simulink model "CompleteModel"  (R2023a)
settings: Solver=VariableStepAuto  StartTime=0.0  StopTime=10.0  RelTol=1e-3
undefined symbols (not defined in the file): Axle1D, AxleIn, Body, Body_Axle2, Brakes_Axle2_None, Chassis_Axle2, Damper, Damper_Basics, Init, Left, Linear, None, Power, Right, Sedan_Hamba_Parts, ShaftA1, ShaftA2, Spring, Spring_Basics, Vehicle, Visual, X, Y, Z
libraries: sm_lib x272, sm_car_lib x96, fl_lib x69, nesl_utility x51, Driveshaft_ShaftsAll x4, Steer_Rack x3, Differential_Systems x2, sdl_lib x2, Linkage_DW_B x2, AntiRollBar_Simple x2, Power_Components x2, Aero_Coefficients x1
(part 1 of 13)
settings Model: Creator=AXIGUEA  LastModifiedBy=AXIGUEA

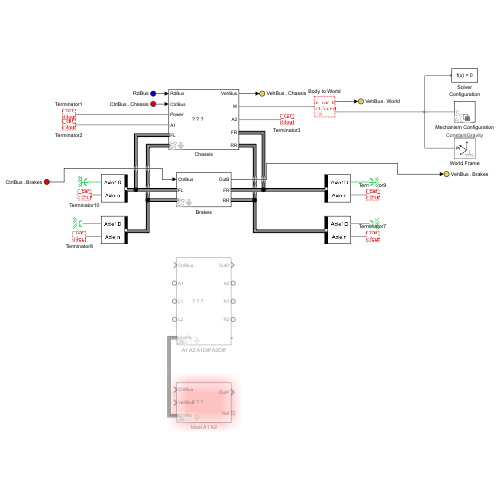
[thumbnail: Simulink's stored preview of the top-level diagram]
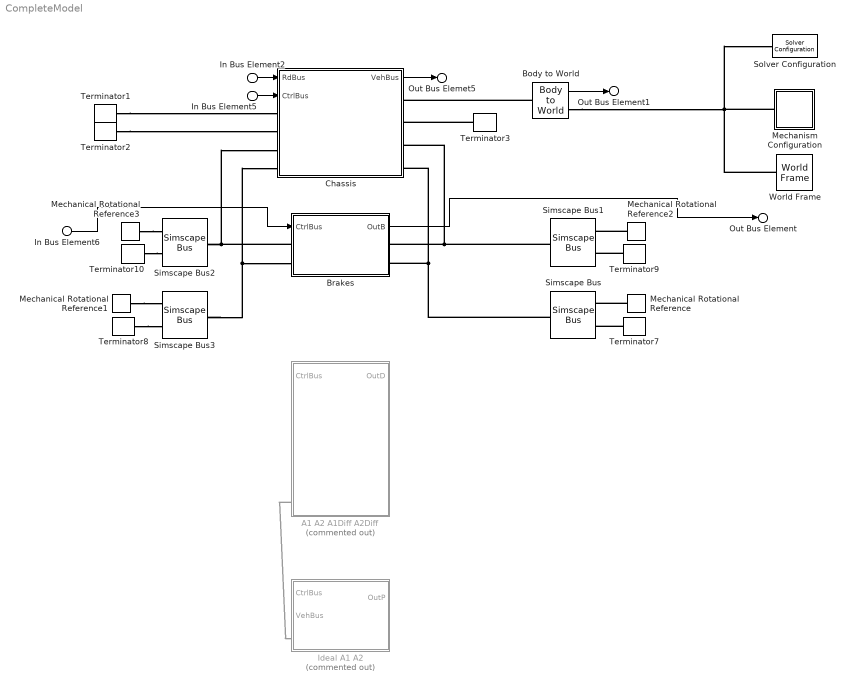
== system CompleteModel ==
  In Bus Element2 : Inport  PortName=RdBus
  In Bus Element5 : Inport  Port=2  PortName=CtrlBus  Element=Chassis
  In Bus Element6 : Inport  Port=2  PortName=CtrlBus  Element=Brakes
  A1 A2 A1Diff A2Diff : Subsystem  Tag=PublishSubsystem  Commented=on  AncestorBlock=Driveline_Axle2_A1_A2_A1Diff_A2Diff/A1 A2 A1Diff A2Diff  VariantControl=A1_A2_A1Diff_A2Diff  mask(Driveline, Two-Axle, Two Input Shaft){InitTriggerDropdown=1}
      mask prompts: InitTriggerDropdown "Initialization Trigger Dropdown"
      mask help: Models two-axle drivelines with differentials on front and rear axles.
      mask init:
      | curblk = gcb;
      | 
      | % Trigger Mask Initialization for 
      | % variant subsystems below this level
      | sm_car_lib_maskInitTrigger(curblk)
      settings: LibrarySourceBlock=Driveline_Axle2_A1_A2_A1Diff_A2Diff/A1 A2 A1Diff A2Diff
      mask TypeOptions InitTriggerDropdown: 0 | 1
      mask Display: image('sm_car_vehicle_driveline_axle2_a1_a2_a1diff_a2diff_IMAGE.png');
  Body to World : sm_car_lib/Body/Body to World  Init=Init.Chassis  SpecifyPosTarget=on
  Brakes : Subsystem  Tag=PublishSubsystem  AncestorBlock=Brakes_Axle2_None/None  VariantControl=None  mask(Brake System Placeholder){}
      mask help: Empty subsystem, used as a variant that omits braking system.
      settings: LibrarySourceBlock=Brakes_Axle2_None/None
  Chassis : Subsystem  Tag=PublishSubsystem  AncestorBlock=Chassis_Axle2/Chassis  VariantControl=Chassis  mask(Chassis){Chassis=Vehicle.Chassis, Init=Init, InitTriggerDropdown=1, mask_image_name=sm_car_vehicle_chassis_hamba_IMAGE.png}
      mask prompts: Chassis "Vehicle Parameters"; Init "Initial Values"; InitTriggerDropdown "Initialization Trigger Dropdown"; mask_image_name "Mask Image (string)"
      mask help: Models vehicle chassis, with suspension, body, tires, springs, and dampers.
      mask init:
      | curblk = gcb;
      | 
      | % Trigger Mask Initialization for 
      | % variant subsystems below this level
      | sm_car_lib_maskInitTrigger(curblk)
      settings: LibrarySourceBlock=Chassis_Axle2/Chassis
      mask Help: web('sm_car_doc_chassis.html')
      mask TypeOptions InitTriggerDropdown: 0 | 1
      mask Display:
      | % Get image from BodyGeometry.class
      | % (active choice for Body Geometry subsystem)
      | temp_veh_bg_class = lower(get_param([gcb '/Body/Body Geometry'],'LabelModeActiveChoice'));
      | 
      | imagestr = (['sm_car_chassis_' temp_veh_bg_class '.png']);
      | if(~exist(imagestr))
      |     imagestr = ['sm_car_chassis_default.png'];
      | end
      | 
      | image(imagestr);
  Ideal A1 A2 : Subsystem  Commented=on  AncestorBlock=Power_Shaft2_Ideal_A1_A2/Ideal A1 A2  VariantControl=Ideal_A1_A2  mask(Two Ideal Motors, Axles 1 and 2){motor_ts_a1=Power.ActuatorCutoffA1.Value, motor_ts_a2=Power.ActuatorCutoffA2.Value}
      mask prompts: motor_ts_a1 "Axle 1 Motor Cutoff Frequency (Hz)"; motor_ts_a2 "Axle 2 Motor Cutoff Frequency (Hz)"
      mask help: Models two ideal motors connected to first and second axles in vehicle driveline.
      settings: LibrarySourceBlock=Power_Shaft2_Ideal_A1_A2/Ideal A1 A2
      mask Display: image('sm_car_vehicle_power_ideal2motor_IMAGE.png');
  Mechanical Rotational Reference{,1..3} (4 alike) : fl_lib/Mechanical/Rotational Elements/Mechanical Rotational Reference
  Mechanism Configuration : Subsystem  AncestorBlock=sm_car_lib/Environment/CarWorldConfig/Mechanism Configuration  Variant=on  VariantControlMode=label  VariantControl=Choice  LabelModeActiveChoice=ConstantGravity
      settings: AttributesFormatString=%<LabelModeActiveChoice>  LibrarySourceBlock=sm_car_lib/Environment/CarWorldConfig/Mechanism Configuration
      mask Display: disp(' ');
  Simscape Bus{,1..3} (4 alike) : SimscapeBus  HierarchyStrings=Axle1D;AxleIn
  Solver Configuration : nesl_utility/Solver Configuration  PhysicalDomain=network_engine_domain  SubClassName=solver  LeftPortType=input  RightPortType=generic  Tones=[]  Harmonics=[]  SimulateNoise=off  Profile=off  UseLocalSampling=off  EnableSwitchedLinearOptims=on  FrequencyDomain=off  UseCCode=off  RelTol=0.001  AbsTol=1e-06  MinStep=1e-09  ToWorkspace=off  RevertToSquareIcSolve=off  NumHomotopyIterations=100  PhasorMode=off  PhasorModeNumHarmonics=1  ConsistencySolver=NEWTON_FTOL  IndexReductionMethod=DerivativeReplacement  DoDC=off  ResidualTolerance=1e-9  ConsistencyTolSource=GLOBAL  ConsistencyAbsTol=0.001  ConsistencyRelTol=0.001  ConsistencyTolFactor=0.001  UseLocalSolver=on  LocalSolverChoice=NE_BACKWARD_EULER_ADVANCER  ResolveIndetEquations=on  FunctionEvalNumThread=1  LocalSolverSampleTime=0.005  DoFixedCost=on  MaxNonlinIter=3  MaxModeIter=2  ComputeImpulses=off  ImpulseIterations=2  LinearAlgebra=Sparse  LinearAlgebraNumThread=0  EquationFormulation=NE_TIME_EF  DelaysMemoryBudget=1024  AutomaticFiltering=on  FilteringTimeConstant=0.001  PartitionStorageMethod=AS_NEEDED  PartitionMemoryBudget=1024  PartitionMethod=FAST
  Terminator{1..3,7..10} (7 alike) : sm_car_lib/Utilities/Terminator  SystemSampleTime=-1  VariantActivationTime=update diagram  Latency=0  AutoFrameSizeCalculation=off
  World Frame : sm_lib/Frames and Transforms/World Frame
  Out Bus Element1 : Outport  VectorParamsAs1DForOutWhenUnconnected=off  PortName=VehBus  Element=World
  Out Bus Elemet5 : Outport  VectorParamsAs1DForOutWhenUnconnected=off  PortName=VehBus  Element=Chassis
  Out Bus Element : Outport  VectorParamsAs1DForOutWhenUnconnected=off  PortName=VehBus  Element=Brakes
  wires:
  Body to World/1 -> Out Bus Element1/1
  Chassis/1(VehBus) -> Out Bus Elemet5/1
  In Bus Element2/1 -> Chassis/1(RdBus)
  In Bus Element5/1 -> Chassis/2(CtrlBus)
  In Bus Element6/1 -> Brakes/1(CtrlBus)
  Brakes/1(OutB) -> Out Bus Element/1
  connections:
  Mechanical Rotational Reference/LConn1 -- Simscape Bus/LConn1
  Terminator7/RConn1 -- Simscape Bus/LConn2
  Terminator8/RConn1 -- Simscape Bus3/LConn2
  Mechanical Rotational Reference1/LConn1 -- Simscape Bus3/LConn1
  Terminator9/RConn1 -- Simscape Bus1/LConn2
  Mechanical Rotational Reference2/LConn1 -- Simscape Bus1/LConn1
  Mechanical Rotational Reference3/LConn1 -- Simscape Bus2/LConn1
  Terminator10/RConn1 -- Simscape Bus2/LConn2
  Simscape Bus1/RConn1 -- Brakes/RConn1 -- Chassis/RConn3
  Simscape Bus/RConn1 -- Brakes/RConn2 -- Chassis/RConn4
  Simscape Bus2/RConn1 -- Brakes/LConn1 -- Chassis/LConn3
  Simscape Bus3/RConn1 -- Brakes/LConn2 -- Chassis/LConn4
  Body to World/LConn1 -- Chassis/RConn1
  Terminator3/RConn1 -- Chassis/RConn2
  Terminator1/RConn1 -- Chassis/LConn1
  Terminator2/RConn1 -- Chassis/LConn2
  Mechanism Configuration/RConn1 -- Solver Configuration/RConn1 -- Body to World/RConn1 -- World Frame/RConn1
  A1 A2 A1Diff A2Diff/LConn4 -- Ideal A1 A2/LConn1

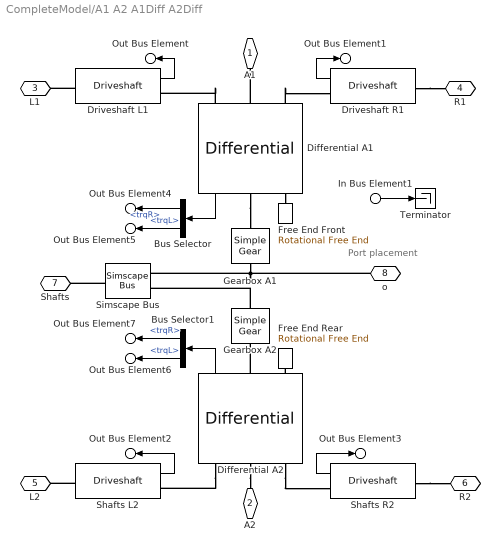
== system CompleteModel/A1 A2 A1Diff A2Diff ==
  note: Port
      | placement
  In Bus Element1 : Inport  PortName=CtrlBus
  Bus Selector : BusSelector  OutputSignals=trqR,trqL
  Bus Selector1 : BusSelector  OutputSignals=trqR,trqL
  Differential A1 : Differential_Systems/Differential  VariantControl=Variant1  LabelModeActiveChoice=Gear1DShafts3D  Differential=Driveline.DifferentialA1  VariantLabel=Driveline.DifferentialA1.class.Value  InitTriggerDropdown=1
      settings: AttributesFormatString=%<ActiveVariant>
  Differential A2 : Differential_Systems/Differential  VariantControl=Variant1  LabelModeActiveChoice=Gear1DShafts1D  Differential=Driveline.DifferentialA2  VariantLabel=Driveline.DifferentialA2.class.Value  InitTriggerDropdown=1
      settings: AttributesFormatString=%<ActiveVariant>
  Driveshaft L1 : Driveshaft_ShaftsAll/Driveshaft  VariantControl=Variant1  LabelModeActiveChoice=Shaft3D  popup_leftRight=Left  Driveshaft=Driveline.DriveshaftL1  VariantLabel=Driveline.DriveshaftL1.class.Value  InitTriggerDropdown=1
      settings: AttributesFormatString=%<ActiveVariant>
  Driveshaft R1 : Driveshaft_ShaftsAll/Driveshaft  VariantControl=Variant1  LabelModeActiveChoice=Shaft3D  popup_leftRight=Right  Driveshaft=Driveline.DriveshaftR1  VariantLabel=Driveline.DriveshaftR1.class.Value  InitTriggerDropdown=1
      settings: AttributesFormatString=%<ActiveVariant>
  Free End Front : fl_lib/Mechanical/Rotational Elements/Rotational Free End  w_specify=off  w_priority=None  w=0 rad/s  w_nominal_specify=off  w_nominal_unit=rad/s  w_nominal_value=1
  Free End Rear : fl_lib/Mechanical/Rotational Elements/Rotational Free End  w_specify=off  w_priority=None  w=0 rad/s  w_nominal_specify=off  w_nominal_unit=rad/s  w_nominal_value=1
  Gearbox A1 : sdl_lib/Gears/Simple Gear  ratio=Driveline.GearboxA1.ratio.Value  rotation_direction=3-2*(1)  friction_model=1  T_noload=0.1 N*m  T_nom=5 N*m  efficiency_nom=0.8  efficiency=0.8  temperature_TLU=[280, 300, 320] K  load_TLU=[1, 5, 10] N*m  efficiency_TLU=[.95, .9, .85]  efficiency_TLU2=[.85, .8, .75; .95, .9, .85; .85, .8, .7]  w_thr=0.01 rad/s  pwr_thr=0.001 W  enable_backlash=false  hardstop_model=simscape.enum.hardstop.smooth  backlash_distance=1e-3 mm  r_base=0.1 m  transition=1e-4 mm  backlash_stiffness=1e7 N/m  backlash_damping=1e6 N*s/m  coeff_rest=0  v_tol=0.001 m/s  f_tol=0 N  mu_visc=[0, 0] N*m/(rad/s)  enable_faults=0  efficiency_fault=0.05  external_fault=simscape.enum.onoff.off  temporal_fault=0  fault_time=5 s  fault_angles=pi / 12 rad  report_fault=(1)-1  thermal_mass=50 J/K  temperature_specify=off  temperature_priority=High  temperature=300 K  temperature_nominal_specify=off  temperature_nominal_unit=K  temperature_nominal_value=1  x_backlash_specify=off  x_backlash_priority=None  x_backlash=0 mm  x_backlash_nominal_specify=off  x_backlash_nominal_unit=mm  x_backlash_nominal_value=1  f_hardstop_specify=off  f_hardstop_priority=None  f_hardstop=0 N  f_hardstop_nominal_specify=off  f_hardstop_nominal_unit=N  f_hardstop_nominal_value=1  v_backlash_specify=off  v_backlash_priority=None  v_backlash=0 m/s  v_backlash_nominal_specify=off  v_backlash_nominal_unit=m/s  v_backlash_nominal_value=1
  Gearbox A2 : sdl_lib/Gears/Simple Gear  ratio=Driveline.GearboxA2.ratio.Value  rotation_direction=3-2*(1)  friction_model=1  T_noload=0.1 N*m  T_nom=5 N*m  efficiency_nom=0.8  efficiency=0.8  temperature_TLU=[280, 300, 320] K  load_TLU=[1, 5, 10] N*m  efficiency_TLU=[.95, .9, .85]  efficiency_TLU2=[.85, .8, .75; .95, .9, .85; .85, .8, .7]  w_thr=0.01 rad/s  pwr_thr=0.001 W  enable_backlash=false  hardstop_model=simscape.enum.hardstop.smooth  backlash_distance=1e-3 mm  r_base=0.1 m  transition=1e-4 mm  backlash_stiffness=1e7 N/m  backlash_damping=1e6 N*s/m  coeff_rest=0  v_tol=0.001 m/s  f_tol=0 N  mu_visc=[0, 0] N*m/(rad/s)  enable_faults=0  efficiency_fault=0.05  external_fault=simscape.enum.onoff.off  temporal_fault=0  fault_time=5 s  fault_angles=pi / 12 rad  report_fault=(1)-1  thermal_mass=50 J/K  temperature_specify=off  temperature_priority=High  temperature=300 K  temperature_nominal_specify=off  temperature_nominal_unit=K  temperature_nominal_value=1  x_backlash_specify=off  x_backlash_priority=None  x_backlash=0 mm  x_backlash_nominal_specify=off  x_backlash_nominal_unit=mm  x_backlash_nominal_value=1  f_hardstop_specify=off  f_hardstop_priority=None  f_hardstop=0 N  f_hardstop_nominal_specify=off  f_hardstop_nominal_unit=N  f_hardstop_nominal_value=1  v_backlash_specify=off  v_backlash_priority=None  v_backlash=0 m/s  v_backlash_nominal_specify=off  v_backlash_nominal_unit=m/s  v_backlash_nominal_value=1
  Shafts L2 : Driveshaft_ShaftsAll/Driveshaft  VariantControl=Variant1  LabelModeActiveChoice=Shaft1D  popup_leftRight=Left  Driveshaft=Driveline.DriveshaftL2  VariantLabel=Driveline.DriveshaftL2.class.Value  InitTriggerDropdown=1
      settings: AttributesFormatString=%<ActiveVariant>
  Shafts R2 : Driveshaft_ShaftsAll/Driveshaft  VariantControl=Variant1  LabelModeActiveChoice=Shaft1D  popup_leftRight=Right  Driveshaft=Driveline.DriveshaftR2  VariantLabel=Driveline.DriveshaftR2.class.Value  InitTriggerDropdown=1
      settings: AttributesFormatString=%<ActiveVariant>
  Simscape Bus : SimscapeBus  HierarchyStrings=ShaftA1;ShaftA2
  Terminator : Terminator
  A1 : PMIOPort  Side=Left
  A2 : PMIOPort  Port=2  Side=Right
  L1 : PMIOPort  Port=3  Side=Left
  R1 : PMIOPort  Port=4  Side=Right
  L2 : PMIOPort  Port=5  Side=Left
  R2 : PMIOPort  Port=6  Side=Right
  Shafts : PMIOPort  Port=7  Side=Left
  o : PMIOPort  Port=8  Side=Right
  Out Bus Element6 : Outport  VectorParamsAs1DForOutWhenUnconnected=off  PortName=OutD  Element=MDriveshaftL2
  Out Bus Element7 : Outport  VectorParamsAs1DForOutWhenUnconnected=off  PortName=OutD  Element=MDriveshaftR2
  Out Bus Element4 : Outport  VectorParamsAs1DForOutWhenUnconnected=off  PortName=OutD  Element=MDriveshaftR1
  Out Bus Element5 : Outport  VectorParamsAs1DForOutWhenUnconnected=off  PortName=OutD  Element=MDriveshaftL1
  Out Bus Element : Outport  VectorParamsAs1DForOutWhenUnconnected=off  PortName=OutD  Element=anDriveshaftL1
  Out Bus Element1 : Outport  VectorParamsAs1DForOutWhenUnconnected=off  PortName=OutD  Element=anDriveshaftR1
  Out Bus Element2 : Outport  VectorParamsAs1DForOutWhenUnconnected=off  PortName=OutD  Element=anDriveshaftL2
  Out Bus Element3 : Outport  VectorParamsAs1DForOutWhenUnconnected=off  PortName=OutD  Element=anDriveshaftR2
  wires:
  In Bus Element1/1 -> Terminator/1
  Bus Selector/2 -> Out Bus Element5/1  "<trqL>"
  Bus Selector/1 -> Out Bus Element4/1  "<trqR>"
  Differential A2/1 -> Bus Selector1/1
  Bus Selector1/2 -> Out Bus Element6/1  "<trqL>"
  Bus Selector1/1 -> Out Bus Element7/1  "<trqR>"
  Differential A1/1 -> Bus Selector/1
  Shafts R2/1 -> Out Bus Element3/1
  Shafts L2/1 -> Out Bus Element2/1
  Driveshaft L1/1 -> Out Bus Element/1
  Driveshaft R1/1 -> Out Bus Element1/1
  connections:
  Simscape Bus/RConn1 -- Shafts/RConn1
  Differential A2/RConn1 -- Gearbox A2/RConn1
  Differential A2/LConn1 -- Shafts L2/RConn1
  Differential A2/LConn3 -- Shafts R2/RConn1
  Shafts L2/LConn1 -- L2/RConn1
  Shafts R2/LConn1 -- R2/RConn1
  Differential A1/RConn1 -- Gearbox A1/RConn1
  Differential A2/LConn2 -- A2/RConn1
  Differential A1/LConn2 -- A1/RConn1
  Driveshaft L1/LConn1 -- L1/RConn1
  Driveshaft R1/LConn1 -- R1/RConn1
  Differential A1/LConn3 -- Driveshaft R1/RConn1
  Differential A1/LConn1 -- Driveshaft L1/RConn1
  Differential A1/RConn2 -- Free End Front/LConn1
  Differential A2/RConn2 -- Free End Rear/LConn1
  Gearbox A1/LConn1 -- o/RConn1 -- Simscape Bus/LConn1
  Gearbox A2/LConn1 -- Simscape Bus/LConn2

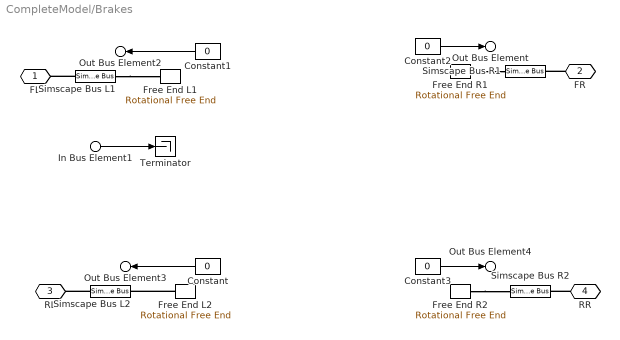
== system CompleteModel/Brakes ==
  In Bus Element1 : Inport  PortName=CtrlBus
  Constant{,1..3} (4 alike) : Constant  Value=0
  Free End L1 : fl_lib/Mechanical/Rotational Elements/Rotational Free End  w_specify=off  w_priority=None  w=0 rad/s  w_nominal_specify=off  w_nominal_unit=rad/s  w_nominal_value=1
  Free End L2 : fl_lib/Mechanical/Rotational Elements/Rotational Free End  w_specify=off  w_priority=None  w=0 rad/s  w_nominal_specify=off  w_nominal_unit=rad/s  w_nominal_value=1
  Free End R1 : fl_lib/Mechanical/Rotational Elements/Rotational Free End  w_specify=off  w_priority=None  w=0 rad/s  w_nominal_specify=off  w_nominal_unit=rad/s  w_nominal_value=1
  Free End R2 : fl_lib/Mechanical/Rotational Elements/Rotational Free End  w_specify=off  w_priority=None  w=0 rad/s  w_nominal_specify=off  w_nominal_unit=rad/s  w_nominal_value=1
  Simscape Bus L1 : SimscapeBus  HierarchyStrings=Axle1D
  Simscape Bus L2 : SimscapeBus  HierarchyStrings=Axle1D
  Simscape Bus R1 : SimscapeBus  HierarchyStrings=Axle1D
  Simscape Bus R2 : SimscapeBus  HierarchyStrings=Axle1D
  Terminator : Terminator
  FL : PMIOPort  Side=Left
  FR : PMIOPort  Port=2  Side=Right
  RL : PMIOPort  Port=3  Side=Left
  RR : PMIOPort  Port=4  Side=Right
  Out Bus Element2 : Outport  VectorParamsAs1DForOutWhenUnconnected=off  PortName=OutB  Element=MBrakeL1
  Out Bus Element : Outport  VectorParamsAs1DForOutWhenUnconnected=off  PortName=OutB  Element=MBrakeR1
  Out Bus Element3 : Outport  VectorParamsAs1DForOutWhenUnconnected=off  PortName=OutB  Element=MBrakeL2
  Out Bus Element4 : Outport  VectorParamsAs1DForOutWhenUnconnected=off  PortName=OutB  Element=MBrakeR2
  wires:
  Constant3/1 -> Out Bus Element4/1
  Constant/1 -> Out Bus Element3/1
  Constant2/1 -> Out Bus Element/1
  Constant1/1 -> Out Bus Element2/1
  In Bus Element1/1 -> Terminator/1
  connections:
  Free End R2/LConn1 -- Simscape Bus R2/LConn1
  Free End L2/LConn1 -- Simscape Bus L2/LConn1
  Free End R1/LConn1 -- Simscape Bus R1/LConn1
  Simscape Bus L1/LConn1 -- Free End L1/LConn1
  Simscape Bus L1/RConn1 -- FL/RConn1
  Simscape Bus L2/RConn1 -- RL/RConn1
  RR/RConn1 -- Simscape Bus R2/RConn1
  FR/RConn1 -- Simscape Bus R1/RConn1

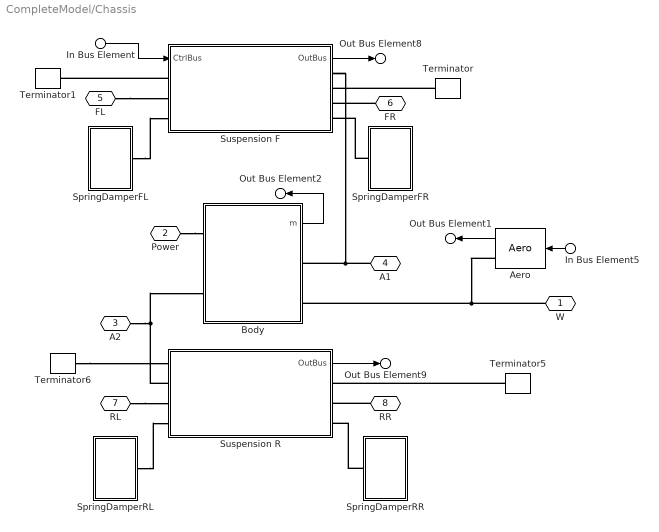
== system CompleteModel/Chassis ==
  In Bus Element5 : Inport  PortName=RdBus  Element=fWindCar
  In Bus Element : Inport  Port=2  PortName=CtrlBus  Element=SuspA1
  Aero : Aero_Coefficients/Aero  CL=Chassis.Aero.CL.Value  CD=Chassis.Aero.CD.Value  rho=Chassis.Aero.rho_air.Value  A=Chassis.Aero.ARef.Value  sCentreOfPressure=Chassis.Aero.sPressureCentre.Value  clr_hp=Visual.hp.clr  opc_hp=Visual.hp.opc  rad_hp=Visual.hp.rad
  Body : Subsystem  AncestorBlock=Body_Axle2/Body  mask(Body){hp_mount_a1=Chassis.Body.sAxle1.Value, hp_mount_a2=Chassis.Body.sAxle2.Value, hp_mount_power=Chassis.Body.sPower.Value, hp_chassis_cg=Chassis.Body.sCG.Value, hp_mount_hitchf=Chassis.Body.sHitchF.Value, hp_mount_hitchr=Chassis.Body.sHitchR.Value, chassis_mass=Chassis.Body.m.Value, chassis_inertia=Chassis.Body.J.Value, clr_chassis_hp_cg=Visual.hp.clr, opc_chassis_hp_cg=Visual.hp.opc, size_chassis_hp_cg=Visual.hp.rad, BodyGeometry=Chassis.Body.BodyGeometry, Passenger=Chassis.Body.Passenger, BodyLoad=Chassis.Body.BodyLoad, InitTriggerDropdown=1}
      mask prompts: hp_mount_power "HP Power [xyz] (m)"; hp_chassis_cg "Chassis CG [xyz] (m)"; hp_mount_hitchf "Hitch Front [xyz] (m)"; hp_mount_hitchr "Hitch Rear [xyz] (m)"; chassis_mass "Mass (kg)"; chassis_inertia "Inertia [Ixx Iyy Izz]"; BodyGeometry "BodyGeometry (structure)"; Passenger "Passenger (structure)"; BodyLoad "BodyLoad (structure)"; InitTriggerDropdown "Initialization Trigger Dropdown"
      mask help: Vehicle body mass, inertia, and geometry.
      mask init:
      | curblk = gcb;
      | 
      | % Trigger Mask Initialization for 
      | % variant subsystems below this level
      | sm_car_lib_maskInitTrigger(curblk)
      settings: LibrarySourceBlock=Body_Axle2/Body
      mask TypeOptions hp_mount_a1:
      | Transform
      | Mount A1/TranslationCartesianOffset
      mask TypeOptions hp_mount_a2:
      | Transform
      | Mount A2/TranslationCartesianOffset
      mask TypeOptions hp_mount_power:
      | Transform
      | Power Mount/TranslationCartesianOffset
      mask TypeOptions hp_chassis_cg:
      | Transform
      | Body CG/TranslationCartesianOffset
      mask TypeOptions hp_mount_hitchf:
      | Transform
      | Front Hitch/TranslationCartesianOffset
      mask TypeOptions hp_mount_hitchr:
      | Transform
      | Rear Hitch/TranslationCartesianOffset
      mask TypeOptions chassis_mass:
      | Body Mass
      | and Inertia/Mass
      mask TypeOptions chassis_inertia:
      | Body Mass
      | and Inertia/MomentsOfInertia
      mask TypeOptions clr_chassis_hp_cg:
      | Body Mass
      | and Inertia/GraphicDiffuseColor | Vis HP Mount A1/GraphicDiffuseColor | Vis HP Hitch/GraphicDiffuseColor
      mask TypeOptions opc_chassis_hp_cg:
      | Body Mass
      | and Inertia/GraphicOpacity | Vis HP Mount A1/GraphicOpacity | Vis HP Hitch/GraphicOpacity
      mask TypeOptions size_chassis_hp_cg:
      | Body Mass
      | and Inertia/SphereRadius | Vis HP Mount A1/SphereRadius | Vis HP Hitch/SphereRadius
      mask TypeOptions InitTriggerDropdown: 0 | 1
      mask DialogControl cont_chassis Prompt: Chassis
      mask DialogControl text_chassis_mount_hp_blank Prompt: [xyz] (m)
      mask DialogControl text_chassis_a1 Prompt: Axle 1
      mask DialogControl text_chassis_a2 Prompt: Axle 2
      mask DialogControl text_chassis_hp_mount Prompt: HP Mount
      mask DialogControl cont_chassis_vis Prompt: Visualization
      mask DialogControl text_chassis_vis_clr Prompt: Color [RGB]
      mask DialogControl text_chassis_vis_opc Prompt: Opacity (0-1)
      mask DialogControl text_chassis_vis_size Prompt: Size [xyz] (m)
      mask DialogControl text_chassis_vis_hp Prompt: Hardpoints
      mask DialogControl cont_body_geometry Prompt: Body
      mask Display:
      | % Get image from BodyGeometry.class
      | % (active choice for Body Geometry subsystem)
      | temp_veh_bg_class = lower(get_param([gcb '/Body Geometry'],'LabelModeActiveChoice'));
      | 
      | imagestr = (['sm_car_body_' temp_veh_bg_class '.png']);
      | if(~exist(imagestr))
      |     imagestr = ['sm_car_body_default.png'];
      | end
      | 
      | image(imagestr);
  SpringDamperFL : Subsystem
  SpringDamperFR : Subsystem
  SpringDamperRL : Subsystem
  SpringDamperRR : Subsystem
  Suspension F : Subsystem  mask{Susp=Chassis.SuspA1, Init=Init.Axle1}
      mask prompts: Susp "Suspension Parameters"; Init "Initial Values"
      mask Display: image('sm_car_vehicle_susp_linkage_IMAGE.png'); % Use "Edit Image" on toolstrip to change.
  Suspension R : Subsystem  mask{Susp=Chassis.SuspA2, Init=Init.Axle2}
      mask prompts: Susp "Suspension Parameters"; Init "Initial Values"
      mask Display: image('sm_car_vehicle_susp_linkage_IMAGE.png'); % Use "Edit Image" on toolstrip to change.
  Terminator{,1,5..6} (4 alike) : sm_car_lib/Utilities/Terminator  SystemSampleTime=-1  VariantActivationTime=update diagram  Latency=0  AutoFrameSizeCalculation=off
  W : PMIOPort  Side=Right
  Power : PMIOPort  Port=2  Side=Left
  A2 : PMIOPort  Port=3  Side=Right
  A1 : PMIOPort  Port=4  Side=Left
  FL : PMIOPort  Port=5  Side=Left
  FR : PMIOPort  Port=6  Side=Right
  RL : PMIOPort  Port=7  Side=Left
  RR : PMIOPort  Port=8  Side=Right
  Out Bus Element2 : Outport  VectorParamsAs1DForOutWhenUnconnected=off  PortName=VehBus  Element=Body
  Out Bus Element1 : Outport  VectorParamsAs1DForOutWhenUnconnected=off  PortName=VehBus  Element=Aero
  Out Bus Element8 : Outport  VectorParamsAs1DForOutWhenUnconnected=off  PortName=VehBus  Element=SuspA1
  Out Bus Element9 : Outport  VectorParamsAs1DForOutWhenUnconnected=off  PortName=VehBus  Element=SuspA2
  wires:
  Body/1(m) -> Out Bus Element2/1
  Aero/1 -> Out Bus Element1/1
  In Bus Element5/1 -> Aero/1
  In Bus Element/1 -> Suspension F/1(CtrlBus)
  Suspension F/1(OutBus) -> Out Bus Element8/1
  Suspension R/1(OutBus) -> Out Bus Element9/1
  connections:
  Terminator6/RConn1 -- Suspension R/LConn1
  Terminator5/RConn1 -- Suspension R/RConn1
  Suspension F/LConn1 -- Terminator1/RConn1
  Power/RConn1 -- Body/LConn1
  Suspension F/RConn1 -- A1/RConn1 -- Body/RConn1
  Terminator/RConn1 -- Suspension F/RConn2
  W/RConn1 -- Aero/RConn1 -- Body/RConn2
  FL/RConn1 -- Suspension F/LConn2
  FR/RConn1 -- Suspension F/RConn3
  RL/RConn1 -- Suspension R/LConn3
  RR/RConn1 -- Suspension R/RConn2
  SpringDamperFR/LConn1 -- Suspension F/RConn4
  SpringDamperFL/LConn1 -- Suspension F/LConn3
  SpringDamperRL/LConn1 -- Suspension R/LConn4
  SpringDamperRR/LConn1 -- Suspension R/RConn3
  A2/RConn1 -- Body/LConn2 -- Suspension R/LConn2

== system CompleteModel/Ideal A1 A2 ==
  note: Future: react torque from
      | drive on chassis
  In Bus Element1 : Inport  PortName=CtrlBus  Element=MMotorA1Demand
  In Bus Element2 : Inport  PortName=CtrlBus  Element=MMotorA2Demand
  VehBus : Inport  Port=2
  Mechanical Rotational Reference1 : fl_lib/Mechanical/Rotational Elements/Mechanical Rotational Reference
  Motor Front : TransferFcn  Denominator=[1/motor_ts_a1 1]
  Motor Rear : TransferFcn  Denominator=[1/motor_ts_a2 1]
  Reference Frame : sm_lib/Frames and Transforms/Reference Frame
  Sensing MotorA1 : Power_Components/Sensing Ideal Motor  Commented=on  SystemSampleTime=-1  VariantActivationTime=update diagram  Latency=0  AutoFrameSizeCalculation=off
  Sensing MotorA2 : Power_Components/Sensing Ideal Motor  Commented=on  SystemSampleTime=-1  VariantActivationTime=update diagram  Latency=0  AutoFrameSizeCalculation=off
  Simscape Bus : SimscapeBus  HierarchyStrings=ShaftA1;ShaftA2
  Simulink-PS Converter1 : nesl_utility/Simulink-PS Converter  PhysicalDomain=network_engine_domain  SubClassName=ps_input  LeftPortType=input  RightPortType=output  PseudoPeriodic=off  Frequencies=[]  NoiseDistribution=none  NoiseParameters=[]  Unit=1  AffineConversion=off  FilteringAndDerivatives=provide  SimscapeFilterOrder=1  InputFilterTimeConstant=0.001  UdotUserProvided=0
  Simulink-PS Converter3 : nesl_utility/Simulink-PS Converter  PhysicalDomain=network_engine_domain  SubClassName=ps_input  LeftPortType=input  RightPortType=output  PseudoPeriodic=off  Frequencies=[]  NoiseDistribution=none  NoiseParameters=[]  Unit=1  AffineConversion=off  FilteringAndDerivatives=provide  SimscapeFilterOrder=1  InputFilterTimeConstant=0.001  UdotUserProvided=0
  Terminator : Terminator
  Torque Source A1 : fl_lib/Mechanical/Mechanical Sources/Ideal Torque Source
  Torque Source A2 : fl_lib/Mechanical/Mechanical Sources/Ideal Torque Source
  Shafts : PMIOPort  Side=Left
  Ref : PMIOPort  Port=2  Side=Right
  Out Bus Element4 : Outport  VectorParamsAs1DForOutWhenUnconnected=off  PortName=OutP  Element=MotorA1
  Out Bus Element1 : Outport  VectorParamsAs1DForOutWhenUnconnected=off  PortName=OutP  Element=MotorA2
  wires:
  Motor Rear/1 -> Simulink-PS Converter1/1
  Motor Front/1 -> Simulink-PS Converter3/1
  In Bus Element1/1 -> Motor Front/1
  In Bus Element2/1 -> Motor Rear/1
  VehBus/1 -> Terminator/1
  connections:
  Torque Source A2/LConn1 -- Simscape Bus/LConn2
  Torque Source A1/LConn1 -- Simscape Bus/LConn1
  Ref/RConn1 -- Reference Frame/RConn1
  Shafts/RConn1 -- Simscape Bus/RConn1
  Torque Source A2/RConn2 -- Mechanical Rotational Reference1/LConn1 -- Torque Source A1/RConn2
  Simulink-PS Converter1/RConn1 -- Torque Source A2/RConn1
  Torque Source A1/RConn1 -- Simulink-PS Converter3/RConn1

== system CompleteModel/Mechanism Configuration ==
  Constant Gravity : Subsystem  VariantControl=ConstantGravity
  C : PMIOPort  Side=Right

== system CompleteModel/Chassis/Body ==
  Body Geometry : Subsystem  AncestorBlock=BodyGeometry_Axle2/Body Geometry  Variant=on  VariantControlMode=label  VariantControl=Variant1  LabelModeActiveChoice=CAD_Sedan_Hamba  mask(Variants for Vehicle Body Geometry){BodyGeometry=BodyGeometry, VariantLabel=BodyGeometry.class.Value, InitTriggerDropdown=1}
      mask prompts: VariantLabel "Variant Label"; InitTriggerDropdown "Initialization Trigger Dropdown"
      mask help: Select option and provide parameters for vehicle body geometry. Option is chosen by string provided in Variant Label. The parameters for the selected option is contained in Body Geometry data structure.
      mask init:
      | curblk = gcb;
      | 
      | % Set variant for this block 
      | set_param(curblk,'LabelModeActiveChoice',VariantLabel);
      settings: AttributesFormatString=%<LabelModeActiveChoice>  LibrarySourceBlock=BodyGeometry_Axle2/Body Geometry
      mask TypeOptions InitTriggerDropdown: 0 | 1
      mask Display:
      | % Display same mask as active variant
      | blk = sm_car_lib_activeVariantBlock(gcb);
      | 
      | if(~isempty(blk))
      |     eval(get_param(blk, 'MaskDisplay'));
      | else
      |     disp(' ');
      | end
  Body Mass and Inertia : sm_lib/Body Elements/Spherical Solid  GraphicAmbientColor=[0.15 0.15 0.15 1.0]  BasedOnType=Density  CenterOfMass=[0 0 0]  CenterOfMassUnits=m  GraphicDiffuseColor=clr_chassis_hp_cg  Density=312*0.6  DensityUnits=kg/m^3  DoExposeReferenceFrame=on  GraphicEmissiveColor=[0.0 0.0 0.0 1.0]  ExportEntireGeometry=off  SerializedExposedGeometries=<ExposedGeometries/>  SerializedFrames=<Frames/>  MarkerShape=Sphere  MarkerSize=10  GraphicType=FromGeometry  InertiaType=Custom  Mass=chassis_mass  MassUnits=kg  MomentsOfInertia=chassis_inertia  MomentsOfInertiaUnits=kg*m^2  GraphicOpacity=opc_chassis_hp_cg  ProductsOfInertia=[0 0 0]  ProductsOfInertiaUnits=kg*m^2  GraphicShininess=75  GraphicSpecularColor=[0.5 0.5 0.5 1.0]  SphereRadius=size_chassis_hp_cg  SphereRadiusUnits=m  GraphicVisPropType=SimpleVisualProperties
  Body Sensor : sm_car_lib/Sensors/Body Sensor  offset_body_sensor=[0 0 0]
  Transform Body CG : sm_lib/Frames and Transforms/Rigid Transform  TranslationMethod=Cartesian  TranslationStandardOffset=0  TranslationStandardOffsetUnits=m  TranslationStandardAxis=+Z  TranslationCartesianOffset=hp_chassis_cg  TranslationCartesianOffsetUnits=m  TranslationROffset=0  TranslationROffsetUnits=m  TranslationZOffset=0  TranslationZOffsetUnits=m  TranslationThetaOffset=0  TranslationThetaOffsetUnits=deg  RotationMethod=None  RotationAngleUnits=deg  RotationStandardAxis=+Z  RotationAngle=0.0  RotationArbitraryAxis=[0 0 1]  FollAlignAxisA=+X  BaseAlignAxisA=+Y  FollAlignAxisB=+Y  BaseAlignAxisB=+Z  RotationSequenceAxes=FollowerAxes  RotationSequence=XYX  RotationSequenceAngles=[0 0 0]  RotationSequenceAnglesUnits=deg  RotationMatrix=[1 0 0; 0 1 0; 0 0 1]  Quaternion=[1 0 0 0]
  Transform Mount A1 : sm_lib/Frames and Transforms/Rigid Transform  TranslationMethod=Cartesian  TranslationStandardOffset=0  TranslationStandardOffsetUnits=m  TranslationStandardAxis=+X  TranslationCartesianOffset=hp_mount_a1  TranslationCartesianOffsetUnits=m  TranslationROffset=0  TranslationROffsetUnits=m  TranslationZOffset=0  TranslationZOffsetUnits=m  TranslationThetaOffset=0  TranslationThetaOffsetUnits=deg  RotationMethod=None  RotationAngleUnits=deg  RotationStandardAxis=+Z  RotationAngle=0.0  RotationArbitraryAxis=[0 0 1]  FollAlignAxisA=+X  BaseAlignAxisA=+Y  FollAlignAxisB=+Y  BaseAlignAxisB=+Z  RotationSequenceAxes=FollowerAxes  RotationSequence=XYX  RotationSequenceAngles=[0 0 0]  RotationSequenceAnglesUnits=deg  RotationMatrix=[1 0 0; 0 1 0; 0 0 1]  Quaternion=[1 0 0 0]
  Transform Mount A2 : sm_lib/Frames and Transforms/Rigid Transform  TranslationMethod=Cartesian  TranslationStandardOffset=0  TranslationStandardOffsetUnits=m  TranslationStandardAxis=-X  TranslationCartesianOffset=hp_mount_a2  TranslationCartesianOffsetUnits=m  TranslationROffset=0  TranslationROffsetUnits=m  TranslationZOffset=0  TranslationZOffsetUnits=m  TranslationThetaOffset=0  TranslationThetaOffsetUnits=deg  RotationMethod=None  RotationAngleUnits=deg  RotationStandardAxis=+Z  RotationAngle=0.0  RotationArbitraryAxis=[0 0 1]  FollAlignAxisA=+X  BaseAlignAxisA=+Y  FollAlignAxisB=+Y  BaseAlignAxisB=+Z  RotationSequenceAxes=FollowerAxes  RotationSequence=XYX  RotationSequenceAngles=[0 0 0]  RotationSequenceAnglesUnits=deg  RotationMatrix=[1 0 0; 0 1 0; 0 0 1]  Quaternion=[1 0 0 0]
  Transform Power Mount : sm_lib/Frames and Transforms/Rigid Transform  TranslationMethod=Cartesian  TranslationStandardOffset=0  TranslationStandardOffsetUnits=m  TranslationStandardAxis=+Z  TranslationCartesianOffset=hp_mount_power  TranslationCartesianOffsetUnits=m  TranslationROffset=0  TranslationROffsetUnits=m  TranslationZOffset=0  TranslationZOffsetUnits=m  TranslationThetaOffset=0  TranslationThetaOffsetUnits=deg  RotationMethod=None  RotationAngleUnits=deg  RotationStandardAxis=+Z  RotationAngle=0.0  RotationArbitraryAxis=[0 0 1]  FollAlignAxisA=+X  BaseAlignAxisA=+Y  FollAlignAxisB=+Y  BaseAlignAxisB=+Z  RotationSequenceAxes=FollowerAxes  RotationSequence=XYX  RotationSequenceAngles=[0 0 0]  RotationSequenceAnglesUnits=deg  RotationMatrix=[1 0 0; 0 1 0; 0 0 1]  Quaternion=[1 0 0 0]
  Vis HP Mount A1 : sm_lib/Body Elements/Spherical Solid  GraphicAmbientColor=[0.15 0.15 0.15 1.0]  BasedOnType=Density  CenterOfMass=[0 0 0]  CenterOfMassUnits=m  GraphicDiffuseColor=clr_chassis_hp_cg  Density=312*0.6  DensityUnits=kg/m^3  DoExposeReferenceFrame=on  GraphicEmissiveColor=[0.0 0.0 0.0 1.0]  ExportEntireGeometry=off  SerializedExposedGeometries=<ExposedGeometries/>  SerializedFrames=<Frames/>  MarkerShape=Sphere  MarkerSize=10  GraphicType=FromGeometry  InertiaType=PointMass  Mass=0  MassUnits=kg  MomentsOfInertia=[1 1 1]  MomentsOfInertiaUnits=kg*m^2  GraphicOpacity=opc_chassis_hp_cg  ProductsOfInertia=[0 0 0]  ProductsOfInertiaUnits=kg*m^2  GraphicShininess=75  GraphicSpecularColor=[0.5 0.5 0.5 1.0]  SphereRadius=size_chassis_hp_cg  SphereRadiusUnits=m  GraphicVisPropType=SimpleVisualProperties
  Vis HP Mount A2 : sm_lib/Body Elements/Spherical Solid  GraphicAmbientColor=[0.15 0.15 0.15 1.0]  BasedOnType=Density  CenterOfMass=[0 0 0]  CenterOfMassUnits=m  GraphicDiffuseColor=clr_chassis_hp_cg  Density=312*0.6  DensityUnits=kg/m^3  DoExposeReferenceFrame=on  GraphicEmissiveColor=[0.0 0.0 0.0 1.0]  ExportEntireGeometry=off  SerializedExposedGeometries=<ExposedGeometries/>  SerializedFrames=<Frames/>  MarkerShape=Sphere  MarkerSize=10  GraphicType=FromGeometry  InertiaType=PointMass  Mass=0  MassUnits=kg  MomentsOfInertia=[1 1 1]  MomentsOfInertiaUnits=kg*m^2  GraphicOpacity=opc_chassis_hp_cg  ProductsOfInertia=[0 0 0]  ProductsOfInertiaUnits=kg*m^2  GraphicShininess=75  GraphicSpecularColor=[0.5 0.5 0.5 1.0]  SphereRadius=size_chassis_hp_cg  SphereRadiusUnits=m  GraphicVisPropType=SimpleVisualProperties
  A1 : PMIOPort  Side=Right
  Pwr : PMIOPort  Port=2  Side=Left
  W : PMIOPort  Port=3  Side=Right
  A2 : PMIOPort  Port=4  Side=Left
  Out Bus Element1 : Outport  VectorParamsAs1DForOutWhenUnconnected=off  PortName=m  Element=CG
  wires:
  Body Sensor/1 -> Out Bus Element1/1
  connections:
  Transform Body CG/LConn1 -- Transform Power Mount/LConn1 -- W/RConn1 -- Transform Mount A1/LConn1 -- Body Geometry/LConn1 -- Transform Mount A2/LConn1
  Body Mass and Inertia/RConn1 -- Body Sensor/LConn1 -- Transform Body CG/RConn1
  Vis HP Mount A1/RConn1 -- Transform Mount A1/RConn1 -- A1/RConn1
  A2/RConn1 -- Vis HP Mount A2/RConn1 -- Transform Mount A2/RConn1
  Pwr/RConn1 -- Transform Power Mount/RConn1

== system CompleteModel/Chassis/SpringDamperFL ==
  Damper : Subsystem  AncestorBlock=Damper_Basics/Linear  VariantControl=Linear  mask(Linear Damper with Bumpstop){dam_b=Chassis.Damper.Damping.d.Value, hp_dpr_top=Chassis.Damper.Damping.sTop.Value, hp_dpr_bot=Chassis.Damper.Damping.sBottom.Value, bs_lim_upper=Chassis.Damper.Endstop.xMax.Value, bs_lim_lower=Chassis.Damper.Endstop.xMin.Value, bs_k_upper=Chassis.Damper.Endstop.KxMax.Value, bs_k_lower=Chassis.Damper.Endstop.KxMin.Value, bs_b_upper=Chassis.Damper.Endstop.dxMax.Value, bs_b_lower=Chassis.Damper.Endstop.dxMin.Value, bs_region=Chassis.Damper.Endstop.xTransition.Value}
      mask prompts: dam_b "Damper (N/(m/s))"; hp_dpr_top "HP Damper Top [xyz] (m)"; hp_dpr_bot "HP Damper Bottom [xyz] (m)"; bs_region "Transition Region (m)"
      mask help: Linear damper with bumpstop at top and bottom.
      mask init:
      | dam_x0 = norm(hp_dpr_top - hp_dpr_bot);
      settings: LibrarySourceBlock=Damper_Basics/Linear
      mask TypeOptions dam_b: Damper/D
      mask DialogControl text_bumpstop_upper Prompt: Upper
      mask DialogControl text_bumpstop_lower Prompt: Lower
      mask DialogControl text_bumpstop_limit Prompt: Limit (m)
      mask DialogControl text_bumpstop_k Prompt: Stiffness (N/m)
      mask DialogControl text_bumpstop_b Prompt: Damping  (N/(m/s))
  MTRef : fl_lib/Mechanical/Translational Elements/Mechanical Translational Reference
  Spring : Subsystem  AncestorBlock=Spring_Basics/Linear  VariantControl=Linear  mask(Linear Spring){spr_def0=Chassis.Spring.xPreload.Value, spr_k=Chassis.Spring.K.Value, spr_hp_top=Chassis.Spring.sTop.Value, spr_hp_bot=Chassis.Spring.sBottom.Value}
      mask prompts: spr_def0 "Spring Preload (m)"; spr_k "Spring Rate (N/m)"; spr_hp_top "HP Top [xyz] (m)"; spr_hp_bot "HP Bottom [xyz] (m)"
      mask help: Spring with linear stiffness.
      mask init:
      | spr_len0 = norm(spr_hp_top-spr_hp_bot);
      settings: LibrarySourceBlock=Spring_Basics/Linear
  Terminator : Terminator
  Terminator1 : Terminator
  R : PMIOPort  Side=Left
  wires:
  Damper/1(meas) -> Terminator1/1
  Spring/1(meas) -> Terminator/1
  connections:
  Spring/LConn1 -- R/RConn1 -- Damper/LConn1
  Damper/RConn1 -- MTRef/LConn1 -- Spring/RConn1

== system CompleteModel/Chassis/SpringDamperFR ==
  Damper : Subsystem  AncestorBlock=Damper_Basics/Linear  VariantControl=Linear  mask(Linear Damper with Bumpstop){dam_b=Damper.Damping.d.Value, hp_dpr_top=Damper.Damping.sTop.Value, hp_dpr_bot=Damper.Damping.sBottom.Value, bs_lim_upper=Damper.Endstop.xMax.Value, bs_lim_lower=Damper.Endstop.xMin.Value, bs_k_upper=Damper.Endstop.KxMax.Value, bs_k_lower=Damper.Endstop.KxMin.Value, bs_b_upper=Damper.Endstop.dxMax.Value, bs_b_lower=Damper.Endstop.dxMin.Value, bs_region=Damper.Endstop.xTransition.Value}
      mask prompts: dam_b "Damper (N/(m/s))"; hp_dpr_top "HP Damper Top [xyz] (m)"; hp_dpr_bot "HP Damper Bottom [xyz] (m)"; bs_region "Transition Region (m)"
      mask help: Linear damper with bumpstop at top and bottom.
      mask init:
      | dam_x0 = norm(hp_dpr_top - hp_dpr_bot);
      settings: LibrarySourceBlock=Damper_Basics/Linear
      mask TypeOptions dam_b: Damper/D
      mask DialogControl text_bumpstop_upper Prompt: Upper
      mask DialogControl text_bumpstop_lower Prompt: Lower
      mask DialogControl text_bumpstop_limit Prompt: Limit (m)
      mask DialogControl text_bumpstop_k Prompt: Stiffness (N/m)
      mask DialogControl text_bumpstop_b Prompt: Damping  (N/(m/s))
  MTRef : fl_lib/Mechanical/Translational Elements/Mechanical Translational Reference
  Spring : Subsystem  AncestorBlock=Spring_Basics/Linear  VariantControl=Linear  mask(Linear Spring){spr_def0=Spring.xPreload.Value, spr_k=Spring.K.Value, spr_hp_top=Spring.sTop.Value, spr_hp_bot=Spring.sBottom.Value}
      mask prompts: spr_def0 "Spring Preload (m)"; spr_k "Spring Rate (N/m)"; spr_hp_top "HP Top [xyz] (m)"; spr_hp_bot "HP Bottom [xyz] (m)"
      mask help: Spring with linear stiffness.
      mask init:
      | spr_len0 = norm(spr_hp_top-spr_hp_bot);
      settings: LibrarySourceBlock=Spring_Basics/Linear
  Terminator : Terminator
  Terminator1 : Terminator
  R : PMIOPort  Side=Left
  wires:
  Damper/1(meas) -> Terminator1/1
  Spring/1(meas) -> Terminator/1
  connections:
  Spring/LConn1 -- R/RConn1 -- Damper/LConn1
  Damper/RConn1 -- MTRef/LConn1 -- Spring/RConn1

== system CompleteModel/Chassis/SpringDamperRL ==
  Damper : Subsystem  AncestorBlock=Damper_Basics/Linear  VariantControl=Linear  mask(Linear Damper with Bumpstop){dam_b=Damper.Damping.d.Value, hp_dpr_top=Damper.Damping.sTop.Value, hp_dpr_bot=Damper.Damping.sBottom.Value, bs_lim_upper=Damper.Endstop.xMax.Value, bs_lim_lower=Damper.Endstop.xMin.Value, bs_k_upper=Damper.Endstop.KxMax.Value, bs_k_lower=Damper.Endstop.KxMin.Value, bs_b_upper=Damper.Endstop.dxMax.Value, bs_b_lower=Damper.Endstop.dxMin.Value, bs_region=Damper.Endstop.xTransition.Value}
      mask prompts: dam_b "Damper (N/(m/s))"; hp_dpr_top "HP Damper Top [xyz] (m)"; hp_dpr_bot "HP Damper Bottom [xyz] (m)"; bs_region "Transition Region (m)"
      mask help: Linear damper with bumpstop at top and bottom.
      mask init:
      | dam_x0 = norm(hp_dpr_top - hp_dpr_bot);
      settings: LibrarySourceBlock=Damper_Basics/Linear
      mask TypeOptions dam_b: Damper/D
      mask DialogControl text_bumpstop_upper Prompt: Upper
      mask DialogControl text_bumpstop_lower Prompt: Lower
      mask DialogControl text_bumpstop_limit Prompt: Limit (m)
      mask DialogControl text_bumpstop_k Prompt: Stiffness (N/m)
      mask DialogControl text_bumpstop_b Prompt: Damping  (N/(m/s))
  MTRef : fl_lib/Mechanical/Translational Elements/Mechanical Translational Reference
  Spring : Subsystem  AncestorBlock=Spring_Basics/Linear  VariantControl=Linear  mask(Linear Spring){spr_def0=Spring.xPreload.Value, spr_k=Spring.K.Value, spr_hp_top=Spring.sTop.Value, spr_hp_bot=Spring.sBottom.Value}
      mask prompts: spr_def0 "Spring Preload (m)"; spr_k "Spring Rate (N/m)"; spr_hp_top "HP Top [xyz] (m)"; spr_hp_bot "HP Bottom [xyz] (m)"
      mask help: Spring with linear stiffness.
      mask init:
      | spr_len0 = norm(spr_hp_top-spr_hp_bot);
      settings: LibrarySourceBlock=Spring_Basics/Linear
  Terminator : Terminator
  Terminator1 : Terminator
  R : PMIOPort  Side=Left
  wires:
  Damper/1(meas) -> Terminator1/1
  Spring/1(meas) -> Terminator/1
  connections:
  Spring/LConn1 -- R/RConn1 -- Damper/LConn1
  Damper/RConn1 -- MTRef/LConn1 -- Spring/RConn1

== system CompleteModel/Chassis/SpringDamperRR ==
  Damper : Subsystem  AncestorBlock=Damper_Basics/Linear  VariantControl=Linear  mask(Linear Damper with Bumpstop){dam_b=Damper.Damping.d.Value, hp_dpr_top=Damper.Damping.sTop.Value, hp_dpr_bot=Damper.Damping.sBottom.Value, bs_lim_upper=Damper.Endstop.xMax.Value, bs_lim_lower=Damper.Endstop.xMin.Value, bs_k_upper=Damper.Endstop.KxMax.Value, bs_k_lower=Damper.Endstop.KxMin.Value, bs_b_upper=Damper.Endstop.dxMax.Value, bs_b_lower=Damper.Endstop.dxMin.Value, bs_region=Damper.Endstop.xTransition.Value}
      mask prompts: dam_b "Damper (N/(m/s))"; hp_dpr_top "HP Damper Top [xyz] (m)"; hp_dpr_bot "HP Damper Bottom [xyz] (m)"; bs_region "Transition Region (m)"
      mask help: Linear damper with bumpstop at top and bottom.
      mask init:
      | dam_x0 = norm(hp_dpr_top - hp_dpr_bot);
      settings: LibrarySourceBlock=Damper_Basics/Linear
      mask TypeOptions dam_b: Damper/D
      mask DialogControl text_bumpstop_upper Prompt: Upper
      mask DialogControl text_bumpstop_lower Prompt: Lower
      mask DialogControl text_bumpstop_limit Prompt: Limit (m)
      mask DialogControl text_bumpstop_k Prompt: Stiffness (N/m)
      mask DialogControl text_bumpstop_b Prompt: Damping  (N/(m/s))
  MTRef : fl_lib/Mechanical/Translational Elements/Mechanical Translational Reference
  Spring : Subsystem  AncestorBlock=Spring_Basics/Linear  VariantControl=Linear  mask(Linear Spring){spr_def0=Spring.xPreload.Value, spr_k=Spring.K.Value, spr_hp_top=Spring.sTop.Value, spr_hp_bot=Spring.sBottom.Value}
      mask prompts: spr_def0 "Spring Preload (m)"; spr_k "Spring Rate (N/m)"; spr_hp_top "HP Top [xyz] (m)"; spr_hp_bot "HP Bottom [xyz] (m)"
      mask help: Spring with linear stiffness.
      mask init:
      | spr_len0 = norm(spr_hp_top-spr_hp_bot);
      settings: LibrarySourceBlock=Spring_Basics/Linear
  Terminator : Terminator
  Terminator1 : Terminator
  R : PMIOPort  Side=Left
  wires:
  Damper/1(meas) -> Terminator1/1
  Spring/1(meas) -> Terminator/1
  connections:
  Spring/LConn1 -- R/RConn1 -- Damper/LConn1
  Damper/RConn1 -- MTRef/LConn1 -- Spring/RConn1
